simulink model "sfbuilder_movingAverage"  (R2019b)
settings: Solver=VariableStepAuto  StartTime=0.0  StopTime=10.0  RelTol=1e-3
settings Model: Creator=The MathWorks, Inc.  LastModifiedBy=julie
settings DebuggingCC: ArithmeticOperatorsInVariantConditions=warning
settings SFSimCC: SimUseLocalCustomCode=off  CustomCodeUndefinedFunction=UseInterfaceOnly
settings RTWCC: RTWUseLocalCustomCode=off

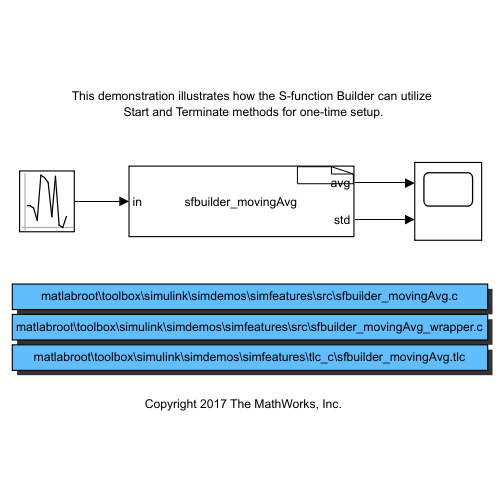
[thumbnail: Simulink's stored preview of the top-level diagram]
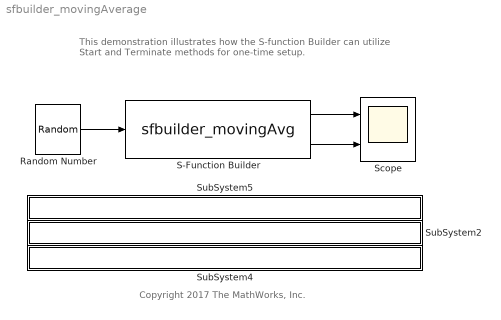
== system sfbuilder_movingAverage ==
  note: This demonstration illustrates how the S-function Builder can utilize
      |  Start and Terminate methods for one-time setup.
  note: Copyright 2017 The MathWorks, Inc.
  Random Number : RandomNumber  SampleTime=0.1
  S-Function Builder : S-Function  InitFcn=try, set_param(gcb,'FunctionName','sfbuilder_movingAvg'), end  FunctionName=sfbuilder_movingAvg  Parameters=5  SFunctionModules=sfbuilder_movingAvg_wrapper  SFunctionDeploymentMode=off  EnableBusSupport=off  mask(S-Function Builder){}
      mask help: Simulink:masks:SFunctionBuilder_MD
      mask init:
      | val = [[.9  0.75 0.75 1 1 .9 .9 1]',[1 1 0.75 0.75 .9 .9 1 .9]'];try , sys = get_param(gcb,'SfunBuilderFcnName');if isempty(sys), sys = get_param(gcb,'FunctionName'); end,catch, sys = get_param(gcb,'FunctionName'); end
      settings: CopyFcn=set_param(gcbh,'LinkStatus','none')  PreSaveFcn=try, set_param(gcb,'FunctionName','sfbuilder_movingAvg'), end  OpenFcn=sfunctionwizard(gcbh)
      mask Display: plot(val(:,1),val(:,2)),disp(sys), port_label('input',1,'in'), port_label('output',1,'avg'), port_label('output',2,'std')
  Scope : Scope  NumInputPorts=2
  SubSystem2 : Subsystem  mask{filename=sfbuilder_movingAvg_wrapper.c}
      mask init:
      | x=sfundemo_maskdisp;
      settings: AttributesFormatString=\n  OpenFcn=sfundemo_openfcn
      mask Display: disp(x);
  SubSystem4 : Subsystem  mask{filename=sfbuilder_movingAvg.tlc}
      mask init:
      | x=sfundemo_maskdisp;
      settings: AttributesFormatString=\n  OpenFcn=sfundemo_openfcn
      mask Display: disp(x);
  SubSystem5 : Subsystem  mask{filename=sfbuilder_movingAvg.c}
      mask init:
      | x=sfundemo_maskdisp;
      settings: AttributesFormatString=\n  OpenFcn=sfundemo_openfcn
      mask Display: disp(x);
  wires:
  S-Function Builder/1 -> Scope/1
  Random Number/1 -> S-Function Builder/1
  S-Function Builder/2 -> Scope/2

== system sfbuilder_movingAverage/SubSystem2 ==

== system sfbuilder_movingAverage/SubSystem4 ==

== system sfbuilder_movingAverage/SubSystem5 ==
